simulink model "ParadigmPresenterStandardModel_gNautilus"  (R2017a)
settings: Solver=FixedStepDiscrete  StartTime=0.0  StopTime=inf  FixedStep=1/250  RelTol=1e-3  EnableMultiTasking=on
model workspace (MAT data in the model file):
  cfg_native : struct (value not decoded)
  en_add_channels = 1
  host_ip = 2130706433
  host_port = 50223
  local_ip = 2130706433
  local_port = 50224
  num_en_channels = 8
  num_samples = 1
  sample_rate = 250
  serial_number = 'NR-2018.09.02'
undefined symbols (not defined in the file or in its folder): groupMap, NR
libraries: gtecHighspeedLib x5, gNautilusLib x1
settings Model: ModifiedByFormat=g.tec  Creator=g.tec medical engineering  LastModifiedBy=g.tec
settings DataIOCC: LimitDataPoints=on  SaveFormat=Array
settings OptimizationCC: LifeSpan=inf
settings DebuggingCC: SFUnexpectedBacktrackingDiag=warning  SFNoUnconditionalDefaultTransitionDiag=warning  SFExecutionAtInitializationDiag=none
settings HardwareCC: ProdBitPerPointer=32  ProdBitPerSizeT=32  ProdBitPerPtrDiffT=32  ProdLargestAtomicFloat=None  ProdIntDivRoundTo=Undefined  ProdEndianess=Unspecified  ProdWordSize=32  ProdHWDeviceType=32-bit Generic
settings ModelReferenceCC: PropagateSignalLabelsOutOfModel=off
settings GRTTargetCC: TargetLangStandard=C89/C90 (ANSI)  GeneratePreprocessorConditionals=Disable all
settings ConfigComp: CovMetricSettings=dw  CovHtmlReporting=on  CovSaveCumulativeToWorkspaceVar=on  CovSaveSingleToWorkspaceVar=on  CovExternalEMLEnable=off

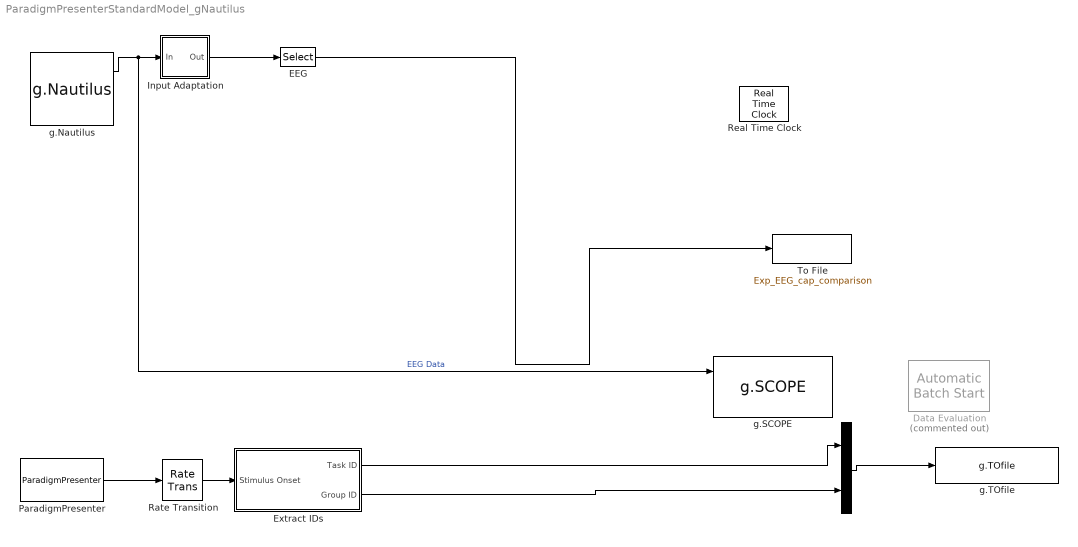
== system ParadigmPresenterStandardModel_gNautilus ==
  "  " : Concatenate
  Data Evaluation : gtecHighspeedLib/Automatic  Batch Start  Commented=on  batch2start='AEP_P300_Evaluation'  nameToFileBlock=empty
      settings: SourceProductName=g.tec Highspeed Library
  EEG : Selector  InputPortWidth=8  IndexOptions=Index vector (dialog)  Indices=[1:8]  OutputSizes=1
  Extract IDs : Subsystem
  Input Adaptation : Subsystem
  ParadigmPresenter : gtecHighspeedLib/ParadigmPresenter  Priority=2  sharedMemoryId=U99Z6EV6EI  bufferSize=000001  sampleRateOrig=000250  stimQuantizationUs=002000  paradigmRootFolder=D:\EEG_caps_comparison_main_folder\EEG_caps_comparison\MotorImagery  logLevel=1  paradigmFiles=\MotorImagery.xml
      settings: SourceProductName=g.tec Highspeed Library
  Rate Transition : RateTransition
  Real Time Clock : gtecHighspeedLib/Real Time Clock  timeprofile=off
      settings: SourceProductName=g.tec Highspeed Library
  To File : ToFile  Filename=Exp_EEG_cap_comparison  MatrixName=y
  g.Nautilus : gNautilusLib/g.Nautilus  Tag=g.Nautilus  Description=Operates a g.Nautilus device and provides acquired data on its outputs.  sample_rate=250  local_ip=2130706433  local_port=50224  host_ip=2130706433  host_port=50223  serial_number=NR-2018.09.02  num_samples=1  num_en_channels=8  add_channels=1
      settings: SourceProductName=g.Nautilus
  g.SCOPE : gtecHighspeedLib/g.SCOPE
      settings: SourceProductName=g.tec Highspeed Library
  g.TOfile : gtecHighspeedLib/g.TOfile  filename=motor_stimuli  varname=y  filesize=1800  blocksize=512  enable=off  save_model=off  patient_data=off  id=ID0000  firstname=John  lastname=Doe  dateofbirth=12.01.2001  sex=FEMALE  hand=MIXED  diagnosis=Diagnosis  medication=Medication Text  comments=any text ...  run=1  session=1
      settings: SourceProductName=g.tec Highspeed Library
  wires:
  "  "/1 -> g.TOfile/1
  ParadigmPresenter/1 -> Rate Transition/1
  Rate Transition/1 -> Extract IDs/1(Stimulus Onset)
  Extract IDs/1(Task ID) -> "  "/1
  Extract IDs/2(Group ID) -> "  "/2
  Input Adaptation/1(Out) -> EEG/1
  g.Nautilus/1 -> g.SCOPE/1, Input Adaptation/1(In)  "EEG Data"
  EEG/1 -> To File/1

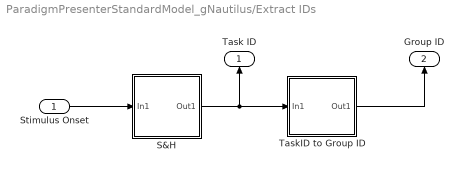
== system ParadigmPresenterStandardModel_gNautilus/Extract IDs ==
  Stimulus Onset : Inport
  S&H : Subsystem
  TaskID to Group ID : Subsystem  InitFcn=|
      | try
      |   taskInfo = evalin('base','taskInfo');
      |   groupMap = taskInfo.Group;
      | catch ME
      |   clear ME;
      |   error('No paradigm loaded!');
      | end
  Task ID : Outport
  Group ID : Outport  Port=2
  wires:
  TaskID to Group ID/1(Out1) -> Group ID/1
  S&H/1(Out1) -> TaskID to Group ID/1(In1), Task ID/1
  Stimulus Onset/1 -> S&H/1(In1)

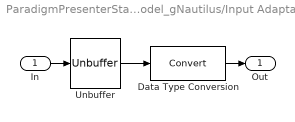
== system ParadigmPresenterStandardModel_gNautilus/Input Adaptation ==
  In : Inport  OutDataTypeStr=single
  Data Type Conversion : DataTypeConversion
  Unbuffer : Unbuffer
  Out : Outport
  wires:
  In/1 -> Unbuffer/1
  Unbuffer/1 -> Data Type Conversion/1
  Data Type Conversion/1 -> Out/1

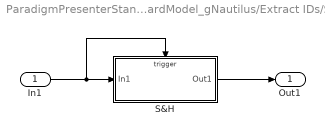
== system ParadigmPresenterStandardModel_gNautilus/Extract IDs/S&H ==
  In1 : Inport
  S&H : Subsystem  TreatAsAtomicUnit=on
  Out1 : Outport
  wires:
  In1/1 -> S&H/Trigger, S&H/1(In1)
  S&H/1(Out1) -> Out1/1

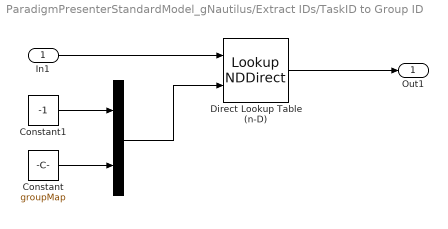
== system ParadigmPresenterStandardModel_gNautilus/Extract IDs/TaskID to Group ID ==
  In1 : Inport
  " " : Concatenate
  Constant : Constant  Value=groupMap
  Constant1 : Constant  Value=-1
  Direct Lookup Table (n-D) : LookupNDDirect  NumberOfTableDimensions=1  TableIsInput=on  Table=[4 5 ;16 19 ]  DiagnosticForOutOfRangeInput=Error
  Out1 : Outport
  wires:
  Direct Lookup Table (n-D)/1 -> Out1/1
  In1/1 -> Direct Lookup Table (n-D)/1
  Constant/1 -> " "/2
  Constant1/1 -> " "/1
  " "/1 -> Direct Lookup Table (n-D)/2

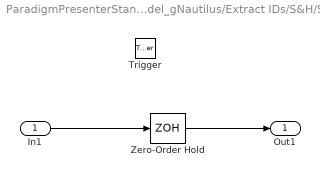
== system ParadigmPresenterStandardModel_gNautilus/Extract IDs/S&H/S&H ==
  In1 : Inport
  Trigger : TriggerPort  VariantControl=Variant
  Zero-Order Hold : ZeroOrderHold  SampleTime=-1
  Out1 : Outport
  wires:
  In1/1 -> Zero-Order Hold/1
  Zero-Order Hold/1 -> Out1/1
